simulink model "Assignment4"  (R2021a)
settings: Solver=VariableStepAuto  StartTime=0.0  StopTime=10.0  RelTol=1e-3
undefined symbols (not defined in the file): A, B, C1
libraries: simulink x1
settings Model: Creator=TITIR  LastModifiedBy=TITIR

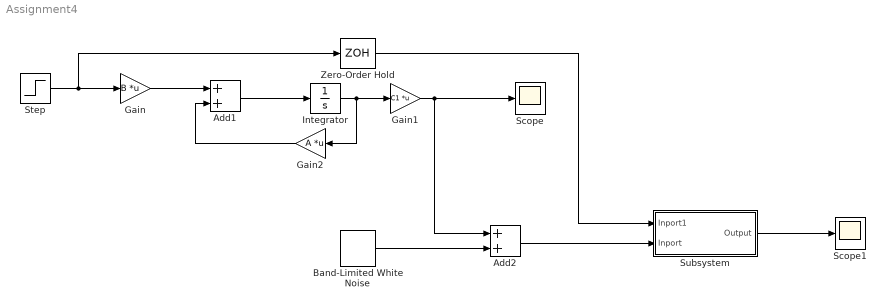
== system Assignment4 ==
  Add1 : Sum
  Add2 : Sum
  Band-Limited White Noise : simulink/Sources/Band-Limited White Noise  Cov=0.005  Ts=0.1  seed=[23341]
  Gain : Gain  Gain=B  Multiplication=Matrix(K*u)
  Gain1 : Gain  Gain=C1  Multiplication=Matrix(K*u)
  Gain2 : Gain  Gain=A  Multiplication=Matrix(K*u)
  Integrator : Integrator  InitialCondition=[0; 0.17; 0; 0]
  Scope : Scope
  Scope1 : Scope
  Step : Step  Time=0  SampleTime=0
  Subsystem : Subsystem
  Zero-Order Hold : ZeroOrderHold  SampleTime=-1
  wires:
  Integrator/1 -> Gain2/1, Gain1/1
  Zero-Order Hold/1 -> Subsystem/1(Inport1)
  Step/1 -> Zero-Order Hold/1, Gain/1
  Band-Limited White Noise/1 -> Add2/2
  Gain2/1 -> Add1/2
  Subsystem/1(Output) -> Scope1/1
  Add1/1 -> Integrator/1
  Gain/1 -> Add1/1
  Gain1/1 -> Add2/1, Scope/1
  Add2/1 -> Subsystem/2(Inport)

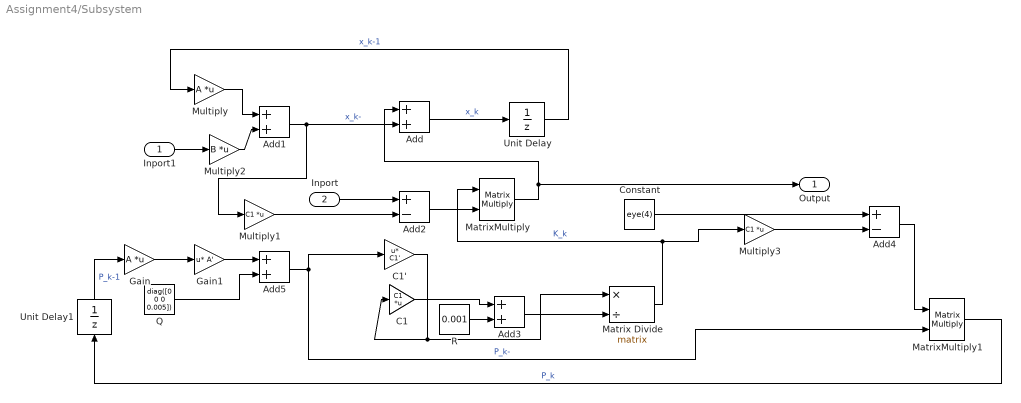
== system Assignment4/Subsystem ==
  Inport1 : Inport
  Inport : Inport  Port=2
  Add{,1,3,5} (4 alike) : Sum
  Add2 : Sum  Inputs=+-
  Add4 : Sum  Inputs=+-
  C1 : Gain  Gain=C1  Multiplication=Matrix(K*u)
  C1' : Gain  Gain=C1'  Multiplication=Matrix(u*K)
  Constant : Constant  Value=eye(4)
  Gain : Gain  Gain=A  Multiplication=Matrix(K*u)
  Gain1 : Gain  Gain=A'  Multiplication=Matrix(u*K)
  Matrix Divide : Product  Inputs=*/  Multiplication=Matrix(*)
  MatrixMultiply : Product  Multiplication=Matrix(*)
  MatrixMultiply1 : Product  Multiplication=Matrix(*)
  Multiply : Gain  Gain=A  Multiplication=Matrix(K*u)
  Multiply1 : Gain  Gain=C1  Multiplication=Matrix(K*u)
  Multiply2 : Gain  Gain=B  Multiplication=Matrix(K*u)
  Multiply3 : Gain  Gain=C1  Multiplication=Matrix(K*u)
  Q : Constant  Value=diag([0 0 0 0.005])
  R : Constant  Value=0.001
  Unit Delay : UnitDelay  SampleTime=-1  HasFrameUpgradeWarning=on
  Unit Delay1 : UnitDelay  SampleTime=-1  HasFrameUpgradeWarning=on
  Output : Outport
  wires:
  Add2/1 -> MatrixMultiply/2
  Q/1 -> Add5/2
  Gain/1 -> Gain1/1
  Unit Delay1/1 -> Gain/1  "P_k-1"
  Gain1/1 -> Add5/1
  R/1 -> Add3/2
  Add5/1 -> MatrixMultiply1/2, C1'/1  "P_k-"
  Inport1/1 -> Multiply2/1
  Constant/1 -> Add4/1
  Unit Delay/1 -> Multiply/1  "x_k-1"
  C1'/1 -> C1/1, Matrix Divide/1
  C1/1 -> Add3/1
  Add4/1 -> MatrixMultiply1/1
  MatrixMultiply1/1 -> Unit Delay1/1  "P_k"
  Multiply1/1 -> Add2/2
  Inport/1 -> Add2/1
  Multiply3/1 -> Add4/2
  Matrix Divide/1 -> MatrixMultiply/1, Multiply3/1  "K_k"
  Multiply/1 -> Add1/1
  Add1/1 -> Multiply1/1, Add/2  "x_k-"
  Add3/1 -> Matrix Divide/2
  MatrixMultiply/1 -> Add/1, Output/1
  Add/1 -> Unit Delay/1  "x_k"
  Multiply2/1 -> Add1/2
